simulink model "sim_model_default"  (R2020b)
settings: Solver=VariableStepAuto  StartTime=0.0  StopTime=10.0  RelTol=1e-3
undefined symbols (not defined in the file): a, b, K
libraries: cstblocks x1
settings Model: Creator=Jonas  LastModifiedBy=Jonas

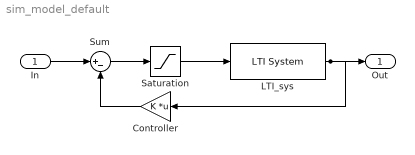
== system sim_model_default ==
  In : Inport
  Controller : Gain  Gain=K  Multiplication=Matrix(K*u)
  LTI_sys : cstblocks/LTI System  sys=lti_sys  IC=x0
  Saturation : Saturate  UpperLimit=b  LowerLimit=a
  Sum : Sum  Inputs=|+-
  Out : Outport
  wires:
  Saturation/1 -> LTI_sys/1
  Controller/1 -> Sum/2
  Sum/1 -> Saturation/1
  LTI_sys/1 -> Controller/1, Out/1
  In/1 -> Sum/1
